simulink model "twoLinks_r"  (Simulink 7.3)
settings: Solver=FixedStepDiscrete  StartTime=0.0  StopTime=inf  FixedStep=Ts  RelTol=1e-3
StartFcn:
  | foundFig=findobj('Tag','trajScope');
  | if ~isempty(foundFig)
  |    close(foundFig);
  | end
undefined symbols (not defined in the file): DiscIntNeverNeededParam, Ts
libraries: simulink x4, dspmtrx3 x2
settings Model: Creator=pattacini  LastModifiedBy=pattacini
settings DataIOCC: LimitDataPoints=off  SaveOutput=off  SignalLogging=off  SaveTime=off  ReturnWorkspaceOutputs=off

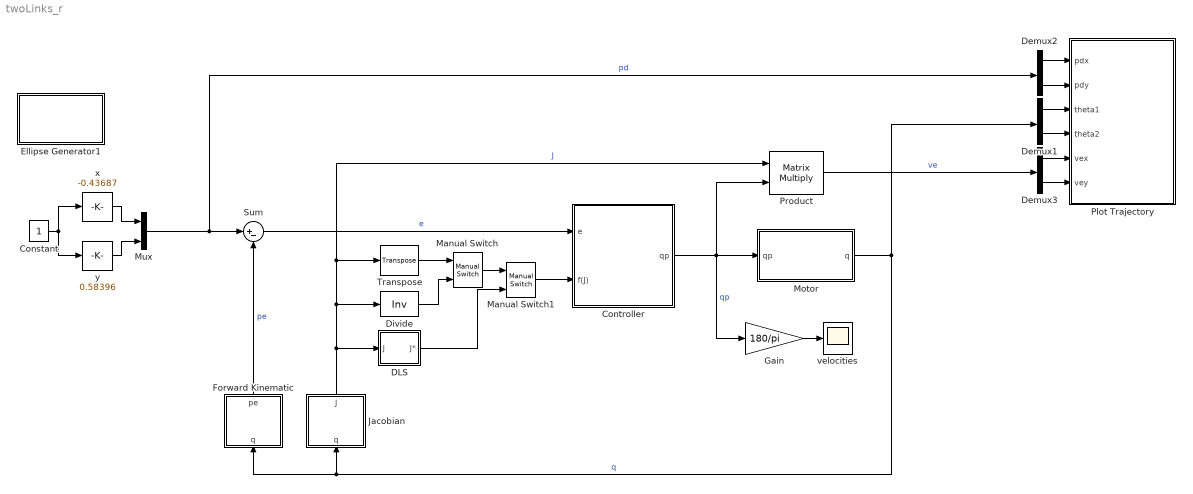
== system twoLinks_r ==
  Constant : Constant
  Controller : Subsystem  mask(Controller settings){K=[1 0; 0 1]}
      mask prompts: K "Gain matrix [2x2]:"
      mask Display: disp('qp=f(J)*K*e');
  DLS : Subsystem  mask(Motor settings){k=0.1}
      mask Display: port_label('input',1,'DLS');
  Demux1 : Demux  Outputs=2
  Demux2 : Demux  Outputs=2
  Demux3 : Demux  Outputs=2
  Divide : Product  Inputs=/  Multiplication=Matrix(*)
  Ellipse Generator1 : Subsystem  mask(Edit sample time){Ts=0.02}
      mask prompts: Ts "Ts [s]:"
      mask init:
      | assignin('base','Ts',Ts);
      mask Display: disp('Edit\nSample Time');
  Forward Kinematic : Subsystem
  Gain : Gain  Gain=180/pi
  Jacobian : Subsystem
  Manual Switch : simulink/Signal Routing/Manual Switch  SystemSampleTime=-1  sw=1  action=0  varsize=off
  Manual Switch1 : simulink/Signal Routing/Manual Switch  SystemSampleTime=-1  sw=0  action=0  varsize=off
  Motor : Subsystem  mask(Motor settings){q0=[pi/4; pi/4]}
      mask prompts: q0 "Initial position [2x1]:"
      mask Display:
      | disp('Motor');
      | port_label('input',1,'qp');
      | port_label('output',1,'q');
  Mux : Mux  Inputs=2
  Plot Trajectory : Stateflow chart  TreatAsAtomicUnit=on
      settings: PermitHierarchicalResolution=ParametersOnly
  Product : Product  Multiplication=Matrix(*)  RndMeth=Zero
  Sum : Sum  Inputs=|+-
  Transpose : dspmtrx3/Transpose  SystemSampleTime=-1  Hermitian=off  overflowFlag=off
  velocities : Scope
      settings: YMin=-65  MaxDataPoints=20000
  x : simulink/Math Operations/Slider Gain  SystemSampleTime=-1  low=-3  gain=-0.43687  high=3
  y : simulink/Math Operations/Slider Gain  SystemSampleTime=-1  low=-3  gain=0.58396  high=3
  wires:
  Jacobian/1(J) -> Transpose/1, Product/1, Divide/1, DLS/1(J)  "J"
  Sum/1 -> Controller/1(e)  "e"
  Forward Kinematic/1(pe) -> Sum/2  "pe"
  Mux/1 -> Sum/1, Demux2/1  "pd"
  Controller/1(qp) -> Motor/1(qp), Product/2, Gain/1  "qp"
  Motor/1(q) -> Demux1/1, Forward Kinematic/1(q), Jacobian/1(q)  "q"
  Demux2/1 -> Plot Trajectory/1(pdx)
  Demux2/2 -> Plot Trajectory/2(pdy)
  Demux1/1 -> Plot Trajectory/3(theta1)
  Demux1/2 -> Plot Trajectory/4(theta2)
  y/1 -> Mux/2
  Constant/1 -> y/1, x/1
  x/1 -> Mux/1
  Demux3/1 -> Plot Trajectory/5(vex)
  Demux3/2 -> Plot Trajectory/6(vey)
  Product/1 -> Demux3/1  "ve"
  Gain/1 -> velocities/1
  Transpose/1 -> Manual Switch/1
  Divide/1 -> Manual Switch/2
  Manual Switch/1 -> Manual Switch1/1
  Manual Switch1/1 -> Controller/2(f(J))
  DLS/1(J*) -> Manual Switch1/2

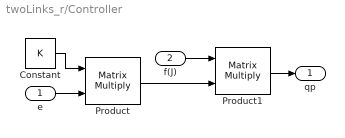
== system twoLinks_r/Controller ==
  e : Inport
  f(J) : Inport  Port=2
  Constant : Constant  Value=K
  Product : Product  Multiplication=Matrix(*)  RndMeth=Zero
  Product1 : Product  Multiplication=Matrix(*)  RndMeth=Zero
  qp : Outport
  wires:
  Product1/1 -> qp/1
  Product/1 -> Product1/2
  f(J)/1 -> Product1/1
  e/1 -> Product/2
  Constant/1 -> Product/1

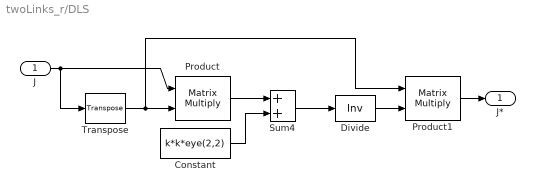
== system twoLinks_r/DLS ==
  J : Inport
  Constant : Constant  Value=k*k*eye(2,2)
  Divide : Product  Inputs=/  Multiplication=Matrix(*)
  Product : Product  Multiplication=Matrix(*)  RndMeth=Zero
  Product1 : Product  Multiplication=Matrix(*)  RndMeth=Zero
  Sum4 : Sum
  Transpose : dspmtrx3/Transpose  SystemSampleTime=-1  Hermitian=off  overflowFlag=off
  J* : Outport
  wires:
  J/1 -> Transpose/1, Product/1
  Transpose/1 -> Product/2, Product1/1
  Product/1 -> Sum4/1
  Sum4/1 -> Divide/1
  Divide/1 -> Product1/2
  Product1/1 -> J*/1
  Constant/1 -> Sum4/2

== system twoLinks_r/Ellipse Generator1 ==

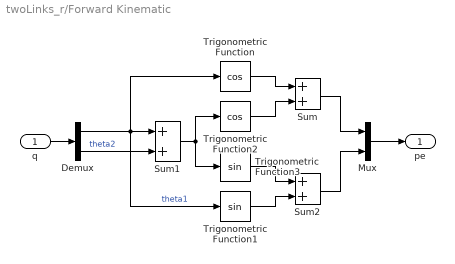
== system twoLinks_r/Forward Kinematic ==
  q : Inport
  Demux : Demux  Outputs=2
  Mux : Mux  Inputs=2
  Sum : Sum
  Sum1 : Sum
  Sum2 : Sum
  Trigonometric Function : Trigonometry  Operator=cos
  Trigonometric Function1 : Trigonometry
  Trigonometric Function2 : Trigonometry  Operator=cos
  Trigonometric Function3 : Trigonometry
  pe : Outport
  wires:
  q/1 -> Demux/1
  Demux/1 -> Trigonometric Function1/1, Trigonometric Function/1, Sum1/1  "theta1"
  Trigonometric Function/1 -> Sum/1
  Sum/1 -> Mux/1
  Mux/1 -> pe/1
  Sum1/1 -> Trigonometric Function2/1, Trigonometric Function3/1
  Trigonometric Function2/1 -> Sum/2
  Demux/2 -> Sum1/2  "theta2"
  Trigonometric Function3/1 -> Sum2/1
  Trigonometric Function1/1 -> Sum2/2
  Sum2/1 -> Mux/2

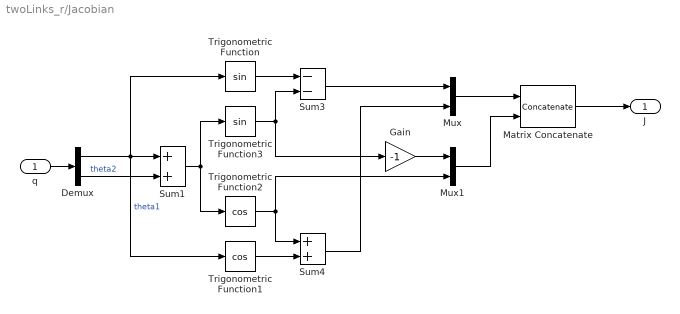
== system twoLinks_r/Jacobian ==
  q : Inport
  Demux : Demux  Outputs=2
  Gain : Gain  Gain=-1
  Matrix Concatenate : Concatenate  Mode=Multidimensional array  ConcatenateDimension=2
  Mux : Mux  Inputs=2
  Mux1 : Mux  Inputs=2
  Sum1 : Sum
  Sum3 : Sum  Inputs=--
  Sum4 : Sum
  Trigonometric Function : Trigonometry
  Trigonometric Function1 : Trigonometry  Operator=cos
  Trigonometric Function2 : Trigonometry  Operator=cos
  Trigonometric Function3 : Trigonometry
  J : Outport
  wires:
  Demux/1 -> Trigonometric Function/1, Trigonometric Function1/1, Sum1/1  "theta1"
  Mux/1 -> Matrix Concatenate/1
  Mux1/1 -> Matrix Concatenate/2
  q/1 -> Demux/1
  Matrix Concatenate/1 -> J/1
  Demux/2 -> Sum1/2  "theta2"
  Trigonometric Function/1 -> Sum3/1
  Sum1/1 -> Trigonometric Function2/1, Trigonometric Function3/1
  Trigonometric Function1/1 -> Sum4/2
  Sum3/1 -> Mux/1
  Sum4/1 -> Mux/2
  Trigonometric Function2/1 -> Sum4/1, Mux1/2
  Trigonometric Function3/1 -> Sum3/2, Gain/1
  Gain/1 -> Mux1/1

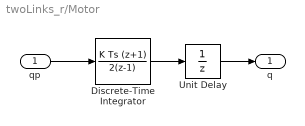
== system twoLinks_r/Motor ==
  qp : Inport
  Discrete-Time Integrator : DiscreteIntegrator  IntegratorMethod=Integration: Trapezoidal  InitialCondition=q0  SampleTime=Ts  ICPrevOutput=DiscIntNeverNeededParam  ICPrevScaledInput=DiscIntNeverNeededParam
  Unit Delay : UnitDelay  X0=q0  SampleTime=-1
  q : Outport
  wires:
  qp/1 -> Discrete-Time Integrator/1
  Discrete-Time Integrator/1 -> Unit Delay/1
  Unit Delay/1 -> q/1

== matlab function Plot Trajectory ==
  data: pdx input double; pdy input double; theta1 input double; theta2 input double; vex input double; vey input double
function PlotTraj(pdx,pdy,theta1,theta2,vex,vey)
% Author: Ugo Pattacini

eml.extrinsic('findobj','get','set','figure','clf',...
              'hold','delete','plot','axis','grid',...
              'hggroup','quiver','drawnow');
          
persistent target;
persistent chain;
persistent velocity;
          
pex=[0;...
    cos(theta1);...
    cos(theta1)+cos(theta1+theta2)];

pey=[0;...
    sin(theta1);...
    sin(theta1)+sin(theta1+theta2)];
          
foundFig=findobj('Tag','trajScope');

if isempty(foundFig)
    fig=figure('Color','white');
    clf(fig);
    set(fig,'Name','Trajectory');
    set(fig,'DoubleBuffer','on','Tag','trajScope');
    set(fig,'Renderer','painters');
    hold('on');
    hax=get(fig,'CurrentAxes');
    set(hax,'DrawMode','fast','Box','off');    
    
    target=plot(hax,pdx,pdy,'bo','MarkerFaceColor','b');

    chain=hggroup;
    h1=plot(hax,pex,pey,'r','LineWidth',3);
    h2=plot(hax,pex(1),pey(1),'ro','MarkerFaceColor','r');
    h3=plot(hax,pex(2),pey(2),'ro','MarkerFaceColor','r');
    h4=plot(hax,pex(3),pey(3),'ro','MarkerFaceColor','r');
    set(h1,'Parent',chain);
    set(h2,'Parent',chain);
    set(h3,'Parent',chain);
    set(h4,'Parent',chain);
    
    velocity=quiver(hax,pex(end),pey(end),vex,vey,'Color','green','LineWidth',2);

    axis([-2.3 2.3 -2.3 2.3]);
    axis('equal');
    grid('on');
else    
    hax=get(foundFig,'CurrentAxes');
end

if ~isempty(chain)
    delete(target);
    delete(chain);
    delete(velocity);
end

% draw the desired point
target=plot(hax,pdx,pdy,'bo','MarkerFaceColor','b');

% draw the link
chain=hggroup;
h1=plot(hax,pex,pey,'r','LineWidth',3);
h2=plot(hax,pex(1),pey(1),'ro','MarkerFaceColor','r');
h3=plot(hax,pex(2),pey(2),'ro','MarkerFaceColor','r');
h4=plot(hax,pex(3),pey(3),'ro','MarkerFaceColor','r');
set(h1,'Parent',chain);
set(h2,'Parent',chain);
set(h3,'Parent',chain);
set(h4,'Parent',chain);

% draw the end-effector velocity in the cartesian space
velocity=quiver(hax,pex(end),pey(end),vex,vey,'Color','green','LineWidth',2);

drawnow;
